simulink model "DSimulator_robot"  (Simulink 7.5)
settings: Solver=ode4  StartTime=0.0  StopTime=10.0  FixedStep=0.01  RelTol=1e-3
undefined symbols (not defined in the file or in its folder): Correct_robot, Dinamic_robot
libraries: roblocks x1
settings Model: Creator=E. Dean  LastModifiedBy=tunc
settings DebuggingCC: StrictBusMsg=Warning

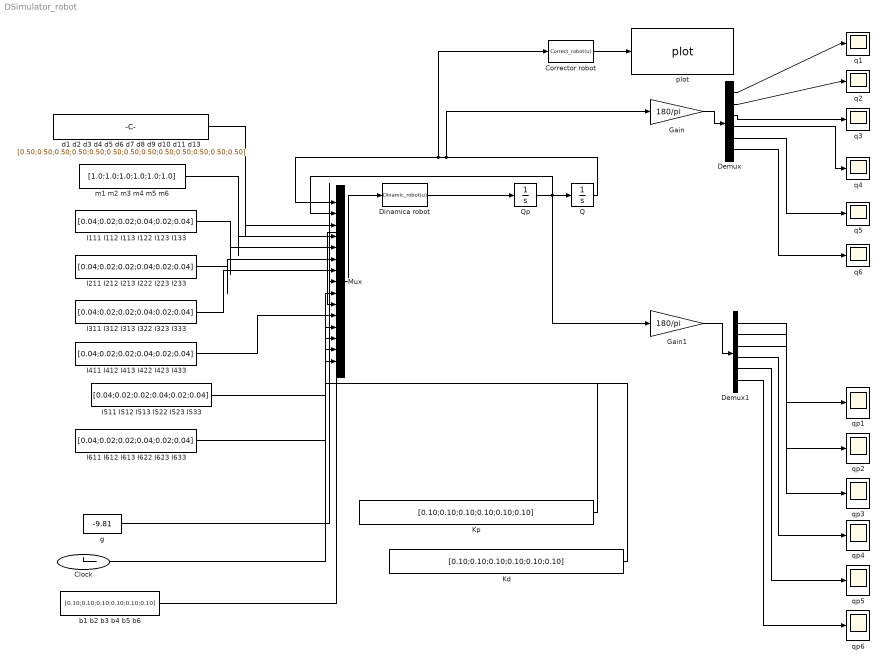
== system DSimulator_robot ==
  Clock : Clock
      settings: Decimation=10
  Corrector robot : MATLABFcn  MATLABFcn=Correct_robot(u)  OutputDimensions=6
  Demux : Demux  Outputs=6
  Demux1 : Demux  Outputs=6
  Dinamica robot : MATLABFcn  MATLABFcn=Dinamic_robot(u)  OutputDimensions=6
  Gain : Gain  Gain=180/pi  ParameterDataType=sfix(16)  ParameterScaling=2^0  OutDataType=sfix(16)  OutScaling=2^0
  Gain1 : Gain  Gain=180/pi  ParameterDataType=sfix(16)  ParameterScaling=2^0  OutDataType=sfix(16)  OutScaling=2^0
  I111 I112 I113 I122 I123 I133 : Constant  Value=[0.04;0.02;0.02;0.04;0.02;0.04]  OutDataType=sfix(16)  OutScaling=2^0
  I211 I212 I213 I222 I223 I233 : Constant  Value=[0.04;0.02;0.02;0.04;0.02;0.04]  OutDataType=sfix(16)  OutScaling=2^0
  I311 I312 I313 I322 I323 I333 : Constant  Value=[0.04;0.02;0.02;0.04;0.02;0.04]  OutDataType=sfix(16)  OutScaling=2^0
  I411 I412 I413 I422 I423 I433 : Constant  Value=[0.04;0.02;0.02;0.04;0.02;0.04]  OutDataType=sfix(16)  OutScaling=2^0
  I511 I512 I513 I522 I523 I533 : Constant  Value=[0.04;0.02;0.02;0.04;0.02;0.04]  OutDataType=sfix(16)  OutScaling=2^0
  I611 I612 I613 I622 I623 I633 : Constant  Value=[0.04;0.02;0.02;0.04;0.02;0.04]  OutDataType=sfix(16)  OutScaling=2^0
  Kd : Constant  Value=[0.10;0.10;0.10;0.10;0.10;0.10]  OutDataType=sfix(16)  OutScaling=2^0
  Kp : Constant  Value=[0.10;0.10;0.10;0.10;0.10;0.10]  OutDataType=sfix(16)  OutScaling=2^0
  Mux : Mux  Inputs=15
  Q : Integrator  InitialCondition=[0;0;0;0;0;0]
  Qp : Integrator  InitialCondition=[0;0;0;0;0;0]
  "b1 b2 b3 b4 b5 b6 " : Constant  Value=[0.10;0.10;0.10;0.10;0.10;0.10]  OutDataType=sfix(16)  OutScaling=2^0
  d1 d2 d3 d4 d5 d6 d7 d8 d9 d10 d11 d13 : Constant  Value=[0.50;0.50;0.50;0.50;0.50;0.50;0.50;0.50;0.50;0.50;0.50;0.50;0.50]  OutDataType=sfix(16)  OutScaling=2^0
  g : Constant  Value=-9.81  OutDataType=sfix(16)  OutScaling=2^0
  "m1 m2 m3 m4 m5 m6 " : Constant  Value=[1.0;1.0;1.0;1.0;1.0;1.0]  OutDataType=sfix(16)  OutScaling=2^0
  plot : roblocks/plot  SystemSampleTime=-1  robot=Robot_robotF
  q{1..6} (6 alike) : Scope
      q1 settings: TimeRange=10  YMin=-6  YMax=4
      q2 settings: TimeRange=10  YMin=-6  YMax=4
      q3 settings: TimeRange=10  YMin=-6  YMax=4
      q4 settings: TimeRange=10  YMin=-6  YMax=4
      q5 settings: TimeRange=10  YMin=-6  YMax=4  SaveName=ScopeData2
      q6 settings: TimeRange=10  YMin=-6  YMax=4  SaveName=ScopeData3
  qp{1..6} (6 alike) : Scope
      qp4 settings: SaveName=ScopeData4
      qp5 settings: SaveName=ScopeData5
      qp6 settings: SaveName=ScopeData6
  wires:
  Qp/1 -> Q/1, Gain1/1, Mux/2
  Mux/1 -> Dinamica robot/1
  Q/1 -> Gain/1, Mux/1, Corrector robot/1
  Gain/1 -> Demux/1
  Demux/1 -> q1/1
  Demux/2 -> q2/1
  Demux/3 -> q3/1
  Gain1/1 -> Demux1/1
  Demux1/1 -> qp1/1
  Demux1/2 -> qp2/1
  Demux1/3 -> qp3/1
  d1 d2 d3 d4 d5 d6 d7 d8 d9 d10 d11 d13/1 -> Mux/3
  "m1 m2 m3 m4 m5 m6 "/1 -> Mux/4
  I111 I112 I113 I122 I123 I133/1 -> Mux/5
  I211 I212 I213 I222 I223 I233/1 -> Mux/6
  I311 I312 I313 I322 I323 I333/1 -> Mux/7
  g/1 -> Mux/8
  Clock/1 -> Mux/9
  "b1 b2 b3 b4 b5 b6 "/1 -> Mux/10
  Corrector robot/1 -> plot/1
  Demux/4 -> q4/1
  Demux/5 -> q5/1
  Demux/6 -> q6/1
  Demux1/4 -> qp4/1
  Demux1/5 -> qp5/1
  Demux1/6 -> qp6/1
  I411 I412 I413 I422 I423 I433/1 -> Mux/11
  I511 I512 I513 I522 I523 I533/1 -> Mux/12
  I611 I612 I613 I622 I623 I633/1 -> Mux/13
  Kp/1 -> Mux/14
  Kd/1 -> Mux/15
  Dinamica robot/1 -> Qp/1
